simulink model "PID"  (R2025b)
settings: Solver=FixedStepAuto  StartTime=0.0  StopTime=10  FixedStep=0.002  RelTol=1e-3
undefined symbols (not defined in the file or in its folder): DiscIntNeverNeededParam, dspblkCoreblockFVToolHelper, gcbh
libraries: simulink x1
settings Model: Creator=flipp  LastModifiedBy=flipp

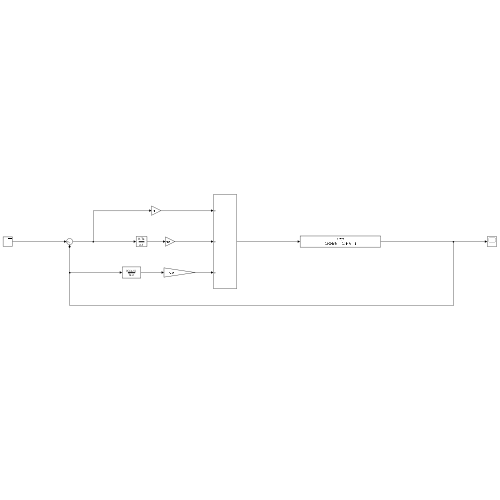
[thumbnail: Simulink's stored preview of the top-level diagram]
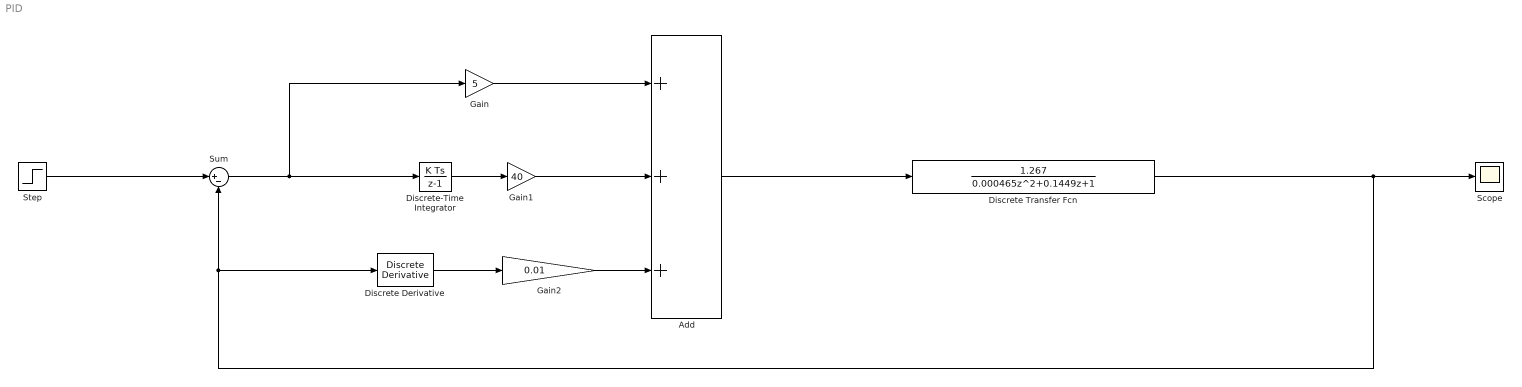
== system PID ==
  Add : Sum  Inputs=+++
  Discrete Transfer Fcn : DiscreteTransferFcn  LoadFcn=dspblkCoreblockFVToolHelper(gcbh,'load');  Numerator=[1.267]  Denominator=[0.000465 0.1449 1]  InitialStates=0.002
      settings: CopyFcn=dspblkCoreblockFVToolHelper(gcbh,'copy');  DeleteFcn=dspblkCoreblockFVToolHelper(gcbh,'close');  ModelCloseFcn=dspblkCoreblockFVToolHelper(gcbh,'close');  PreSaveFcn=dspblkCoreblockFVToolHelper(gcbh,'presave');  PostSaveFcn=dspblkCoreblockFVToolHelper(gcbh,'postsave');  CloseFcn=dspblkCoreblockFVToolHelper(gcbh,'close');
  Discrete Derivative : simulink/Discrete/Discrete Derivative  gainval=1.0  ICPrevScaledInput=0.0  OutMin=[]  OutMax=[]  OutDataType=fixdt(1, 16)  OutScaling=2^-10  DoSatur=off
  Discrete-Time Integrator : DiscreteIntegrator  SampleTime=-1  ICPrevOutput=DiscIntNeverNeededParam  ICPrevScaledInput=DiscIntNeverNeededParam
  Gain : Gain  Gain=5
  Gain1 : Gain  Gain=40
  Gain2 : Gain  Gain=0.01
  Scope : Scope
      settings: ActiveDisplayYMinimum=-47660.604606803987  ActiveDisplayYMaximum=45773.543493804682
  Step : Step  After=10  SampleTime=0
  Sum : Sum  Inputs=|+-
  wires:
  Step/1 -> Sum/1
  Discrete Transfer Fcn/1 -> Scope/1, Sum/2, Discrete Derivative/1
  Gain/1 -> Add/1
  Discrete Derivative/1 -> Gain2/1
  Gain1/1 -> Add/2
  Gain2/1 -> Add/3
  Sum/1 -> Discrete-Time Integrator/1, Gain/1
  Add/1 -> Discrete Transfer Fcn/1
  Discrete-Time Integrator/1 -> Gain1/1
